simulink model "sm_metronome_sync_lots"  (R2026a)
settings: Solver=ode23t  StopTime=5.52*20  MaxStep=1e-2  AbsTol=1e-3  EnableMultiTasking=on
PreLoadFcn:
  | sm_metronome_sync_param
undefined symbols (not defined in the file): M1, M2, M3, M4, metronome, X, Y, Z
libraries: sm_lib x71, sm_metronome_lib x28, nesl_utility x3
(part 1 of 2)
CloseFcn:
  | try,close(h1_sm_metronome_sync),end
  | clear h1_sm_metronome_sync
  | try,close(h2_sm_metronome_sync),end
  | clear h2_sm_metronome_sync
  | try,close(h3_sm_metronome_sync),end
  | clear h3_sm_metronome_sync
  | try,close(h4_sm_metronome_sync),end
  | clear h4_sm_metronome_sync
  | 
  | 
  | clear simlog_sm_metronome_synch
  | clear logsout_sm_metronome_synch
Description:
  | Metronome Synchronization on Moving Platform, Multiple Rows
  | 
  | Copyright 2022-2026 The MathWorks, Inc.
settings Model: PacingRate=4  Creator=smiller  LastModifiedBy=smiller
settings DataIOCC: SaveFormat=StructureWithTime  SignalLoggingName=logsout_sm_metronome_sync
settings SimscapeCC: SimscapeNominalValues="[{\"value\":\"1\",\"unit\":\"A\"},{\"value\":\"1\",\"unit\":\"bar\"},{\"value\":\"1\",\"unit\":\"cm^2\"},{\"value\":\"1\",\"unit\":\"cm^3/s\"},{\"value\":\"1\",\"unit\":\"kJ/kg\"},{\"value\":\"1\",\"unit\":\"kW\"},{\"value\":\"1\",\"unit\":\"l\"},{\"value\":\"1\",\"unit\":\"N\"},{\"value\":\"1\",\"unit\":\"N*m\"},{\"value\":\"1\",\"unit\":\"V\"}]"  SimscapeLogSimulationStatistics=on  SimscapeLogName=simlog_sm_metronome_sync  SimscapeLogDataHistory=50000.0
settings ExplorerConfigSet: InternalSimMechanicsExplorerSettings="<ExplorerConfiguration><canonicalview>default</canonicalview><AnimationSetting><BasePlaybackSpeed>1.0</BasePlaybackSpeed><PlaybackSpeedFactor>4.0</PlaybackSpeedFactor></AnimationSetting><TilePanel><TileInfo><Tiles Columns=\"1\" Count=\"1\" Rows=\"1\"><Column Weight=\"1\"/><Row Weight=\"1\"/><Tile Height=\"1\" Width=\"1\" X=\"0\" Y=\"0\"/></Tiles></TileInfo><SceneInfo><SceneViewer><BGColor><R>1</R><G>1</G><B>1</B></BGColor><Camera><DoPerspective>off</DoPerspective><Position><X>0.415513055170568968</X><Y>-0.891822656871079644</Y><Z>0.234783488518173544</Z></Position><Center><X>-7.26516311720578896e-05</X><Y>0.00999648581965750446</Y><Z>0.116416456880806499</Z></Center><Up><X>-0.0260602284438559428</X><Y>0.118278053469418776</Y><Z>0.992638487346193754</Z></Up><ViewLimDist>1</ViewLimDist><YLim>0.195572453424284781</YLim><XLim>0.452734022015333248</XLim></Camera></SceneViewer></SceneInfo></TilePanel><MechEditorPanel><Cameras/><GfxPanelCameraMap/><VideoCreator><PlaybackSpeedRatio>1.0</PlaybackSpeedRatio><FrameRate>30</FrameRate><VideoFormat>Motion JPEG AVI</VideoFormat><FrameSize>auto</FrameSize></VideoCreator></MechEditorPanel></ExplorerConfiguration>"

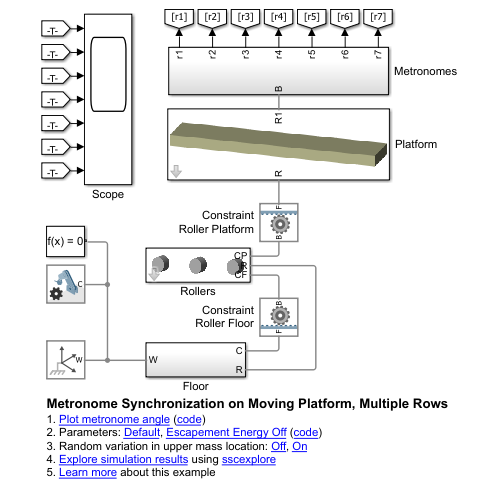
[thumbnail: Simulink's stored preview of the top-level diagram]
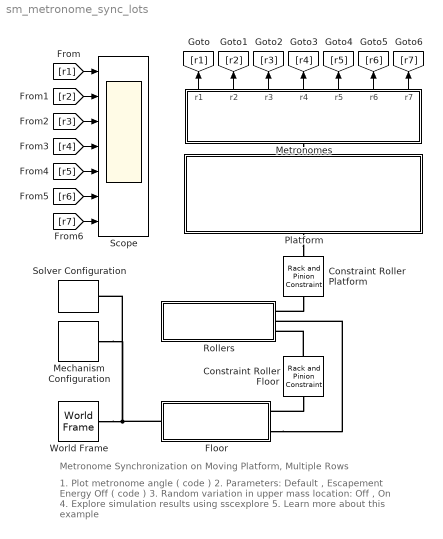
== system sm_metronome_sync_lots ==
  note: Metronome Synchronization on Moving Platform, Multiple Rows
  note: 1. Plot metronome angle ( code )
      | 2. Parameters: Default , Escapement Energy Off ( code )
      | 3. Random variation in upper mass location: Off , On
      | 4. Explore simulation results using sscexplore
      | 5. Learn more about this example
  Constraint Roller Floor : sm_lib/Gears and Couplings/Gears/Rack and Pinion Constraint  PinionRadius=metronome.roller_radius  PinionRadiusUnits=m  SensingForceTorqueDirection=FollowerOnBase  SensingForceTorqueResolutionFrame=BaseFrame  SenseForce=off  SenseTorque=off
  Constraint Roller Platform : sm_lib/Gears and Couplings/Gears/Rack and Pinion Constraint  PinionRadius=metronome.roller_radius  PinionRadiusUnits=m  SensingForceTorqueDirection=FollowerOnBase  SensingForceTorqueResolutionFrame=BaseFrame  SenseForce=off  SenseTorque=off
  Floor : Subsystem
  Mechanism Configuration : sm_lib/Utilities/Mechanism Configuration  UniformGravity=Constant  GravityVector=[0 0 -9.80665]  GravityVectorUnits=m/s^2  LinearizationDelta=0.001  JointModeTransitionNonlinearIterations=2
  Metronomes : Subsystem
  Platform : Subsystem  mask{t_unlock=10, platform_thk=metronome.platform_thickness, roller_rad=metronome.roller_radius}
      mask prompts: t_unlock "Time to Unlock Platform (sec)"; platform_thk "Platform Thickness"; roller_rad "Roller Radius (m)"
      mask Display: image('sm_metronome_sync_platform.png');
  Rollers : Subsystem  mask{roller_rad=metronome.roller_radius, roller_sep=metronome.roller_sep}
      mask prompts: roller_rad "Roller Radius (m)"; roller_sep "Roller Separation (m)"
      mask Display: image('sm_metronome_sync_rollers.png');
  Scope : Scope  NumInputPorts=7
      settings: TimeSpan=5.52/2  ActiveDisplayYMinimum=-1.09829  ActiveDisplayYMaximum=1.09791  DataLoggingVariableName=MetronomeAngles
  Solver Configuration : nesl_utility/Solver Configuration  PhysicalDomain=network_engine_domain  SubClassName=solver  LeftPortType=input  RightPortType=generic  Tones=[]  Harmonics=[]  SimulateNoise=off  Profile=off  UseLocalSampling=off  EnableSwitchedLinearOptims=on  FrequencyDomain=off  UseCCode=off  RelTol=0.001  AbsTol=1e-06  MinStep=1e-09  ToWorkspace=off  RevertToSquareIcSolve=off  NumHomotopyIterations=100  PhasorMode=off  PhasorModeNumHarmonics=1  ConsistencySolver=NEWTON_FTOL  CanonicalOrdering=UNORDERED  OptimizeIntermediates=UNOPTIMIZED  IndexReductionMethod=DerivativeReplacement  DoDC=off  ResidualTolerance=1e-09  ConsistencyTolSource=GLOBAL  ConsistencyAbsTol=0.001  ConsistencyRelTol=0.001  ConsistencyTolFactor=0.001  UseLocalSolver=off  LocalSolverChoice=NE_BACKWARD_EULER_ADVANCER  ResolveIndetEquations=on  FunctionEvalNumThread=1  LocalSolverSampleTime=0.001  DoFixedCost=off  MaxNonlinIter=3  MaxModeIter=2  ComputeImpulses=off  ImpulseIterations=2  LinearAlgebra=Sparse  LinearAlgebraNumThread=0  EquationFormulation=NE_TIME_EF  DelaysMemoryBudget=1024  AutomaticFiltering=on  FilteringTimeConstant=0.001  PartitionStorageMethod=AS_NEEDED  PartitionMemoryBudget=1024  PartitionMethod=FAST  MultibodyUseLocalSolver=off  MultibodyLocalSolverChoice=ODE1  MultibodyLocalSolverSampleTime=0.001
  World Frame : sm_lib/Frames and Transforms/World Frame
  wires:
  Metronomes/1(r1) -> [r1]
  Metronomes/2(r2) -> [r2]
  Metronomes/3(r3) -> [r3]
  Metronomes/4(r4) -> [r4]
  Metronomes/5(r5) -> [r5]
  Metronomes/6(r6) -> [r6]
  Metronomes/7(r7) -> [r7]
  [r1] -> Scope/1
  [r2] -> Scope/2
  [r3] -> Scope/3
  [r4] -> Scope/4
  [r5] -> Scope/5
  [r6] -> Scope/6
  [r7] -> Scope/7
  connections:
  World Frame/RConn1 -- Floor/LConn1 -- Solver Configuration/RConn1 -- Mechanism Configuration/RConn1
  Metronomes/LConn1 -- Platform/RConn1
  Constraint Roller Floor/LConn1 -- Rollers/RConn3
  Floor/RConn2 -- Rollers/RConn2
  Constraint Roller Platform/LConn1 -- Rollers/RConn1
  Constraint Roller Floor/RConn1 -- Floor/RConn1
  Platform/LConn1 -- Constraint Roller Platform/RConn1

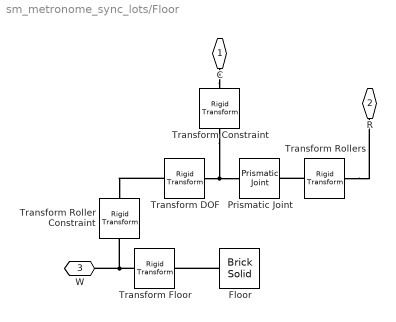
== system sm_metronome_sync_lots/Floor ==
  Floor : sm_lib/Body Elements/Brick Solid  BrickDimensions=[0.75 0.1 0.02]  BrickDimensionsUnits=m  ExportEntireGeometry=off  InertiaType=CalculateFromGeometry  BasedOnType=Density  Density=1000  DensityUnits=kg/m^3  Mass=1  MassUnits=kg  CenterOfMass=[0 0 0]  CenterOfMassUnits=m  MomentsOfInertia=[1 1 1]  MomentsOfInertiaUnits=kg*m^2  ProductsOfInertia=[0 0 0]  ProductsOfInertiaUnits=kg*m^2  GraphicType=FromGeometry  MarkerShape=Sphere  MarkerSize=10  GraphicVisPropType=SimpleVisualProperties  GraphicDiffuseColor=[0.5 0.5 0.5]  GraphicOpacity=1.0  GraphicSpecularColor=[0.5 0.5 0.5 1.0]  GraphicAmbientColor=[0.15 0.15 0.15 1.0]  GraphicEmissiveColor=[0.0 0.0 0.0 1.0]  GraphicShininess=75  DoExposeReferenceFrame=on  SerializedFrames=<Frames/>
  Prismatic Joint : sm_lib/Joints/Prismatic Joint  JointMode=Normal  CompositeWrenchDir=FollowerOnBase  CompositeWrenchFrame=BaseFrame  SenseConstraintForce=off  SenseConstraintTorque=off  SenseTotalForce=off  SenseTotalTorque=off  PositionTargetSpecify=off  PositionTargetPriority=High  PositionTargetValue=0  PositionTargetValueUnits=m  VelocityTargetSpecify=off  VelocityTargetPriority=High  VelocityTargetValue=0  VelocityTargetValueUnits=m/s  EquilibriumPosition=0  EquilibriumPositionUnits=m  SpringStiffness=0  SpringStiffnessUnits=N/m  DampingCoefficient=metronome.platform_damping  DampingCoefficientUnits=N/(m/s)  LowerLimitSpecify=off  LowerLimitBound=-1  LowerLimitBoundUnits=m  LowerLimitStiffness=1e6  LowerLimitStiffnessUnits=N/m  LowerLimitDamping=1e3  LowerLimitDampingUnits=N/(m/s)  LowerLimitTransitionRegionWidth=1e-4  LowerLimitTransitionRegionWidthUnits=m  UpperLimitSpecify=off  UpperLimitBound=1  UpperLimitBoundUnits=m  UpperLimitStiffness=1e6  UpperLimitStiffnessUnits=N/m  UpperLimitDamping=1e3  UpperLimitDampingUnits=N/(m/s)  UpperLimitTransitionRegionWidth=1e-4  UpperLimitTransitionRegionWidthUnits=m  TorqueActuationMode=NoTorque  MotionActuationMode=ComputedMotion  SensePosition=off  SenseVelocity=off  SenseAcceleration=off  SenseTorqueForce=off  SenseLowerLimitTorqueForce=off  SenseUpperLimitTorqueForce=off
  Transform Constraint : sm_lib/Frames and Transforms/Rigid Transform  RotationMethod=StandardAxis  FollAlignAxisA=+X  BaseAlignAxisA=+Y  FollAlignAxisB=+Y  BaseAlignAxisB=+Z  RotationStandardAxis=+Z  RotationAngle=0  RotationAngleUnits=deg  RotationArbitraryAxis=[0 0 1]  RotationSequenceAxes=FollowerAxes  RotationSequence=XYX  RotationSequenceAngles=[0 0 0]  RotationSequenceAnglesUnits=deg  RotationMatrix=[1 0 0; 0 1 0; 0 0 1]  Quaternion=[1 0 0 0]  TranslationMethod=StandardAxis  TranslationCartesianOffset=[0 0 0]  TranslationCartesianOffsetUnits=m  TranslationStandardAxis=+Y  TranslationStandardOffset=-metronome.roller_radius  TranslationStandardOffsetUnits=m  TranslationROffset=0  TranslationROffsetUnits=m  TranslationThetaOffset=0  TranslationThetaOffsetUnits=deg  TranslationZOffset=0  TranslationZOffsetUnits=m
  Transform DOF : sm_lib/Frames and Transforms/Rigid Transform  RotationMethod=StandardAxis  FollAlignAxisA=+X  BaseAlignAxisA=+Y  FollAlignAxisB=+Y  BaseAlignAxisB=+Z  RotationStandardAxis=+Y  RotationAngle=90  RotationAngleUnits=deg  RotationArbitraryAxis=[0 0 1]  RotationSequenceAxes=FollowerAxes  RotationSequence=XYX  RotationSequenceAngles=[0 0 0]  RotationSequenceAnglesUnits=deg  RotationMatrix=[1 0 0; 0 1 0; 0 0 1]  Quaternion=[1 0 0 0]  TranslationMethod=None  TranslationCartesianOffset=[0 0 0]  TranslationCartesianOffsetUnits=m  TranslationStandardAxis=+Z  TranslationStandardOffset=0  TranslationStandardOffsetUnits=m  TranslationROffset=0  TranslationROffsetUnits=m  TranslationThetaOffset=0  TranslationThetaOffsetUnits=deg  TranslationZOffset=0  TranslationZOffsetUnits=m
  Transform Floor : sm_lib/Frames and Transforms/Rigid Transform  RotationMethod=None  FollAlignAxisA=+X  BaseAlignAxisA=+Y  FollAlignAxisB=+Y  BaseAlignAxisB=+Z  RotationStandardAxis=+X  RotationAngle=90  RotationAngleUnits=deg  RotationArbitraryAxis=[0 0 1]  RotationSequenceAxes=FollowerAxes  RotationSequence=XYX  RotationSequenceAngles=[0 0 0]  RotationSequenceAnglesUnits=deg  RotationMatrix=[1 0 0; 0 1 0; 0 0 1]  Quaternion=[1 0 0 0]  TranslationMethod=StandardAxis  TranslationCartesianOffset=[0 0 0]  TranslationCartesianOffsetUnits=m  TranslationStandardAxis=+Z  TranslationStandardOffset=-0.01  TranslationStandardOffsetUnits=m  TranslationROffset=0  TranslationROffsetUnits=m  TranslationThetaOffset=0  TranslationThetaOffsetUnits=deg  TranslationZOffset=0  TranslationZOffsetUnits=m
  Transform Roller Constraint : sm_lib/Frames and Transforms/Rigid Transform  RotationMethod=StandardAxis  FollAlignAxisA=+X  BaseAlignAxisA=+Y  FollAlignAxisB=+Y  BaseAlignAxisB=+Z  RotationStandardAxis=+X  RotationAngle=90  RotationAngleUnits=deg  RotationArbitraryAxis=[0 0 1]  RotationSequenceAxes=FollowerAxes  RotationSequence=XYX  RotationSequenceAngles=[0 0 0]  RotationSequenceAnglesUnits=deg  RotationMatrix=[1 0 0; 0 1 0; 0 0 1]  Quaternion=[1 0 0 0]  TranslationMethod=StandardAxis  TranslationCartesianOffset=[0 0 0]  TranslationCartesianOffsetUnits=m  TranslationStandardAxis=+Z  TranslationStandardOffset=metronome.roller_radius  TranslationStandardOffsetUnits=m  TranslationROffset=0  TranslationROffsetUnits=m  TranslationThetaOffset=0  TranslationThetaOffsetUnits=deg  TranslationZOffset=0  TranslationZOffsetUnits=m
  Transform Rollers : sm_lib/Frames and Transforms/Rigid Transform  RotationMethod=RotationSequence  FollAlignAxisA=+X  BaseAlignAxisA=+Y  FollAlignAxisB=+Y  BaseAlignAxisB=+Z  RotationStandardAxis=+Y  RotationAngle=90  RotationAngleUnits=deg  RotationArbitraryAxis=[0 0 1]  RotationSequenceAxes=FollowerAxes  RotationSequence=YZY  RotationSequenceAngles=[-90 0 0]  RotationSequenceAnglesUnits=deg  RotationMatrix=[1 0 0; 0 1 0; 0 0 1]  Quaternion=[1 0 0 0]  TranslationMethod=None  TranslationCartesianOffset=[0 0 0]  TranslationCartesianOffsetUnits=m  TranslationStandardAxis=+Z  TranslationStandardOffset=0  TranslationStandardOffsetUnits=m  TranslationROffset=0  TranslationROffsetUnits=m  TranslationThetaOffset=0  TranslationThetaOffsetUnits=deg  TranslationZOffset=0  TranslationZOffsetUnits=m
  C : PMIOPort  Side=Right
  R : PMIOPort  Port=2  Side=Right
  W : PMIOPort  Port=3  Side=Left
  connections:
  Floor/RConn1 -- Transform Floor/RConn1
  Transform Rollers/LConn1 -- Prismatic Joint/RConn1
  Transform Floor/LConn1 -- Transform Roller Constraint/LConn1 -- W/RConn1
  Transform DOF/RConn1 -- Transform Constraint/LConn1 -- Prismatic Joint/LConn1
  Transform Rollers/RConn1 -- R/RConn1
  Transform DOF/LConn1 -- Transform Roller Constraint/RConn1
  C/RConn1 -- Transform Constraint/RConn1

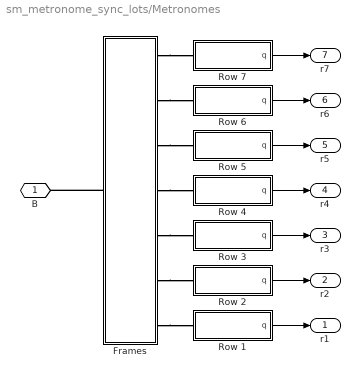
== system sm_metronome_sync_lots/Metronomes ==
  Frames : Subsystem
  Row 1 : Subsystem
  Row 2 : Subsystem
  Row 3 : Subsystem
  Row 4 : Subsystem
  Row 5 : Subsystem
  Row 6 : Subsystem
  Row 7 : Subsystem
  B : PMIOPort  Side=Left
  r1 : Outport
  r2 : Outport  Port=2
  r3 : Outport  Port=3
  r4 : Outport  Port=4
  r5 : Outport  Port=5
  r6 : Outport  Port=6
  r7 : Outport  Port=7
  wires:
  Row 1/1(q) -> r1/1
  Row 2/1(q) -> r2/1
  Row 4/1(q) -> r4/1
  Row 5/1(q) -> r5/1
  Row 3/1(q) -> r3/1
  Row 7/1(q) -> r7/1
  Row 6/1(q) -> r6/1
  connections:
  Frames/RConn3 -- Row 5/LConn1
  Frames/RConn7 -- Row 1/LConn1
  Frames/RConn6 -- Row 2/LConn1
  Frames/RConn5 -- Row 3/LConn1
  Frames/RConn2 -- Row 6/LConn1
  Frames/RConn4 -- Row 4/LConn1
  Frames/RConn1 -- Row 7/LConn1
  Frames/LConn1 -- B/RConn1

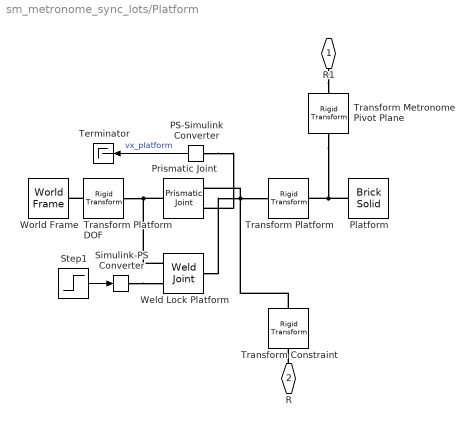
== system sm_metronome_sync_lots/Platform ==
  PS-Simulink Converter : nesl_utility/PS-Simulink Converter  PhysicalDomain=network_engine_domain  SubClassName=ps_output  LeftPortType=input  RightPortType=output  PseudoPeriodic=off  Frequencies=[]  VectorFormat=1-D array  Unit=inherit  AffineConversion=off
  Platform : sm_lib/Body Elements/Brick Solid  BrickDimensions=[0.75 0.75 platform_thk]  BrickDimensionsUnits=m  ExportEntireGeometry=on  InertiaType=CalculateFromGeometry  BasedOnType=Density  Density=10  DensityUnits=kg/m^3  Mass=1  MassUnits=kg  CenterOfMass=[0 0 0]  CenterOfMassUnits=m  MomentsOfInertia=[1 1 1]  MomentsOfInertiaUnits=kg*m^2  ProductsOfInertia=[0 0 0]  ProductsOfInertiaUnits=kg*m^2  GraphicType=FromGeometry  MarkerShape=Sphere  MarkerSize=10  GraphicVisPropType=SimpleVisualProperties  GraphicDiffuseColor=[0.84313726 0.84313726 0.6509804]  GraphicOpacity=1.0  GraphicSpecularColor=[0.5 0.5 0.5 1.0]  GraphicAmbientColor=[0.15 0.15 0.15 1.0]  GraphicEmissiveColor=[0.0 0.0 0.0 1.0]  GraphicShininess=75  DoExposeReferenceFrame=on  SerializedFrames=<Frames/>
  Prismatic Joint : sm_lib/Joints/Prismatic Joint  JointMode=Normal  CompositeWrenchDir=FollowerOnBase  CompositeWrenchFrame=BaseFrame  SenseConstraintForce=off  SenseConstraintTorque=off  SenseTotalForce=off  SenseTotalTorque=off  PositionTargetSpecify=off  PositionTargetPriority=High  PositionTargetValue=0  PositionTargetValueUnits=m  VelocityTargetSpecify=off  VelocityTargetPriority=High  VelocityTargetValue=0  VelocityTargetValueUnits=m/s  EquilibriumPosition=0  EquilibriumPositionUnits=m  SpringStiffness=100*0  SpringStiffnessUnits=N/m  DampingCoefficient=0  DampingCoefficientUnits=N/(m/s)  LowerLimitSpecify=off  LowerLimitBound=-1  LowerLimitBoundUnits=m  LowerLimitStiffness=1e6  LowerLimitStiffnessUnits=N/m  LowerLimitDamping=1e3  LowerLimitDampingUnits=N/(m/s)  LowerLimitTransitionRegionWidth=1e-4  LowerLimitTransitionRegionWidthUnits=m  UpperLimitSpecify=off  UpperLimitBound=1  UpperLimitBoundUnits=m  UpperLimitStiffness=1e6  UpperLimitStiffnessUnits=N/m  UpperLimitDamping=1e3  UpperLimitDampingUnits=N/(m/s)  UpperLimitTransitionRegionWidth=1e-4  UpperLimitTransitionRegionWidthUnits=m  TorqueActuationMode=NoTorque  MotionActuationMode=ComputedMotion  SensePosition=off  SenseVelocity=on  SenseAcceleration=off  SenseTorqueForce=off  SenseLowerLimitTorqueForce=off  SenseUpperLimitTorqueForce=off
  Simulink-PS Converter : nesl_utility/Simulink-PS Converter  PhysicalDomain=network_engine_domain  SubClassName=ps_input  LeftPortType=input  RightPortType=output  PseudoPeriodic=off  Frequencies=[]  NoiseDistribution=none  NoiseParameters=[]  Unit=1  AffineConversion=off  FilteringAndDerivatives=provide  SimscapeFilterOrder=1  InputFilterTimeConstant=0.001  UdotUserProvided=0
  Step1 : Step  Time=t_unlock  FinalValue=-1  SampleTime=0
  Terminator : Terminator
  Transform Constraint : sm_lib/Frames and Transforms/Rigid Transform  RotationMethod=StandardAxis  FollAlignAxisA=+X  BaseAlignAxisA=+Y  FollAlignAxisB=+Y  BaseAlignAxisB=+Z  RotationStandardAxis=+Z  RotationAngle=180  RotationAngleUnits=deg  RotationArbitraryAxis=[0 0 1]  RotationSequenceAxes=FollowerAxes  RotationSequence=XYX  RotationSequenceAngles=[0 0 0]  RotationSequenceAnglesUnits=deg  RotationMatrix=[1 0 0; 0 1 0; 0 0 1]  Quaternion=[1 0 0 0]  TranslationMethod=StandardAxis  TranslationCartesianOffset=[0 0 0]  TranslationCartesianOffsetUnits=m  TranslationStandardAxis=+Y  TranslationStandardOffset=-platform_thk/2  TranslationStandardOffsetUnits=m  TranslationROffset=0  TranslationROffsetUnits=m  TranslationThetaOffset=0  TranslationThetaOffsetUnits=deg  TranslationZOffset=0  TranslationZOffsetUnits=m
  Transform Metronome Pivot Plane : sm_lib/Frames and Transforms/Rigid Transform  RotationMethod=None  FollAlignAxisA=+X  BaseAlignAxisA=+Y  FollAlignAxisB=+Y  BaseAlignAxisB=+Z  RotationStandardAxis=+Z  RotationAngle=0.0  RotationAngleUnits=deg  RotationArbitraryAxis=[0 0 1]  RotationSequenceAxes=FollowerAxes  RotationSequence=XYX  RotationSequenceAngles=[0 0 0]  RotationSequenceAnglesUnits=deg  RotationMatrix=[1 0 0; 0 1 0; 0 0 1]  Quaternion=[1 0 0 0]  TranslationMethod=StandardAxis  TranslationCartesianOffset=[0 0 0]  TranslationCartesianOffsetUnits=m  TranslationStandardAxis=+Z  TranslationStandardOffset=platform_thk/2  TranslationStandardOffsetUnits=m  TranslationROffset=0  TranslationROffsetUnits=m  TranslationThetaOffset=0  TranslationThetaOffsetUnits=deg  TranslationZOffset=0  TranslationZOffsetUnits=m
  Transform Platform : sm_lib/Frames and Transforms/Rigid Transform  RotationMethod=RotationSequence  FollAlignAxisA=+X  BaseAlignAxisA=+Y  FollAlignAxisB=+Y  BaseAlignAxisB=+Z  RotationStandardAxis=+Z  RotationAngle=0.0  RotationAngleUnits=deg  RotationArbitraryAxis=[0 0 1]  RotationSequenceAxes=FollowerAxes  RotationSequence=YZX  RotationSequenceAngles=[90 90 0]  RotationSequenceAnglesUnits=deg  RotationMatrix=[1 0 0; 0 1 0; 0 0 1]  Quaternion=[1 0 0 0]  TranslationMethod=None  TranslationCartesianOffset=[0 0 0]  TranslationCartesianOffsetUnits=m  TranslationStandardAxis=+Z  TranslationStandardOffset=0  TranslationStandardOffsetUnits=m  TranslationROffset=0  TranslationROffsetUnits=m  TranslationThetaOffset=0  TranslationThetaOffsetUnits=deg  TranslationZOffset=0  TranslationZOffsetUnits=m
  Transform Platform DOF : sm_lib/Frames and Transforms/Rigid Transform  RotationMethod=RotationSequence  FollAlignAxisA=+X  BaseAlignAxisA=+Y  FollAlignAxisB=+Y  BaseAlignAxisB=+Z  RotationStandardAxis=+Z  RotationAngle=0.0  RotationAngleUnits=deg  RotationArbitraryAxis=[0 0 1]  RotationSequenceAxes=FollowerAxes  RotationSequence=YZX  RotationSequenceAngles=[90 90 0]  RotationSequenceAnglesUnits=deg  RotationMatrix=[1 0 0; 0 1 0; 0 0 1]  Quaternion=[1 0 0 0]  TranslationMethod=StandardAxis  TranslationCartesianOffset=[0 0 0]  TranslationCartesianOffsetUnits=m  TranslationStandardAxis=+Z  TranslationStandardOffset=roller_rad*2+platform_thk/2  TranslationStandardOffsetUnits=m  TranslationROffset=0  TranslationROffsetUnits=m  TranslationThetaOffset=0  TranslationThetaOffsetUnits=deg  TranslationZOffset=0  TranslationZOffsetUnits=m
  Weld Lock Platform : sm_lib/Joints/Weld Joint  JointMode=ProvidedByInput  CompositeWrenchDir=FollowerOnBase  CompositeWrenchFrame=BaseFrame  SenseConstraintForce=off  SenseConstraintTorque=off  SenseTotalForce=off  SenseTotalTorque=off
  World Frame : sm_lib/Frames and Transforms/World Frame
  R1 : PMIOPort  Side=Right
  R : PMIOPort  Port=2  Side=Left
  wires:
  Step1/1 -> Simulink-PS Converter/1
  PS-Simulink Converter/1 -> Terminator/1  "vx_platform"
  connections:
  Prismatic Joint/RConn1 -- Weld Lock Platform/RConn1 -- Transform Constraint/LConn1 -- Transform Platform/RConn1
  Platform/RConn1 -- Transform Metronome Pivot Plane/LConn1 -- Transform Platform/LConn1
  Transform Platform DOF/RConn1 -- Prismatic Joint/LConn1 -- Weld Lock Platform/LConn1
  Transform Platform DOF/LConn1 -- World Frame/RConn1
  Simulink-PS Converter/RConn1 -- Weld Lock Platform/LConn2
  R1/RConn1 -- Transform Metronome Pivot Plane/RConn1
  PS-Simulink Converter/LConn1 -- Prismatic Joint/RConn2
  R/RConn1 -- Transform Constraint/RConn1

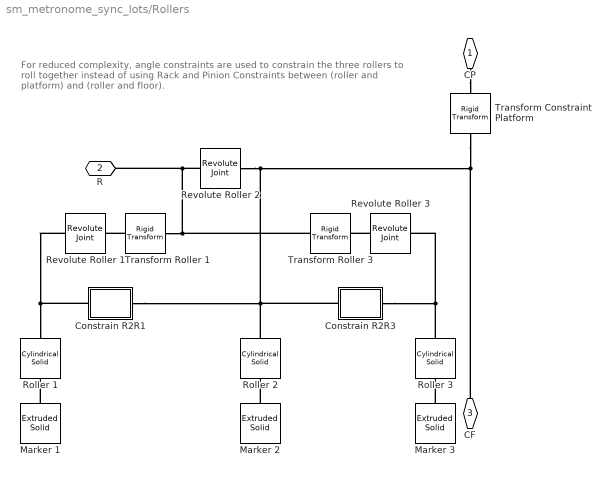
== system sm_metronome_sync_lots/Rollers ==
  note: For reduced complexity, angle constraints are used to constrain the three rollers to roll together instead of using Rack and Pinion Constraints between (roller and platform) and (roller and floor).
  Constrain R2R1 : Subsystem
  Constrain R2R3 : Subsystem
  Marker 1 : sm_lib/Body Elements/Extruded Solid  ExtrusionType=Regular  PolygonNumSides=6  PolygonOuterRadius=roller_rad*0.9  PolygonOuterRadiusUnits=m  ExportEntireGeometry=off  ExtrusionCrossSection=[1 1; -1 1; -1 -1; 1 -1]  ExtrusionCrossSectionUnits=m  ExportConvexHullGeometry=off  ExtrusionLength=1e-3  ExtrusionLengthUnits=m  InertiaType=CalculateFromGeometry  BasedOnType=Mass  Density=1000  DensityUnits=kg/m^3  Mass=0  MassUnits=kg  CenterOfMass=[0 0 0]  CenterOfMassUnits=m  MomentsOfInertia=[1 1 1]  MomentsOfInertiaUnits=kg*m^2  ProductsOfInertia=[0 0 0]  ProductsOfInertiaUnits=kg*m^2  GraphicType=FromGeometry  MarkerShape=Sphere  MarkerSize=10  GraphicVisPropType=SimpleVisualProperties  GraphicDiffuseColor=[0.0 0.2 0.4]  GraphicOpacity=1.0  GraphicSpecularColor=[0.5 0.5 0.5 1.0]  GraphicAmbientColor=[0.15 0.15 0.15 1.0]  GraphicEmissiveColor=[0.0 0.0 0.0 1.0]  GraphicShininess=75  DoExposeReferenceFrame=on  SerializedFrames=<Frames/>
  Marker 2 : sm_lib/Body Elements/Extruded Solid  ExtrusionType=Regular  PolygonNumSides=6  PolygonOuterRadius=roller_rad*0.9  PolygonOuterRadiusUnits=m  ExportEntireGeometry=off  ExtrusionCrossSection=[1 1; -1 1; -1 -1; 1 -1]  ExtrusionCrossSectionUnits=m  ExportConvexHullGeometry=off  ExtrusionLength=1e-3  ExtrusionLengthUnits=m  InertiaType=CalculateFromGeometry  BasedOnType=Mass  Density=1000  DensityUnits=kg/m^3  Mass=0  MassUnits=kg  CenterOfMass=[0 0 0]  CenterOfMassUnits=m  MomentsOfInertia=[1 1 1]  MomentsOfInertiaUnits=kg*m^2  ProductsOfInertia=[0 0 0]  ProductsOfInertiaUnits=kg*m^2  GraphicType=FromGeometry  MarkerShape=Sphere  MarkerSize=10  GraphicVisPropType=SimpleVisualProperties  GraphicDiffuseColor=[0.0 0.2 0.4]  GraphicOpacity=1.0  GraphicSpecularColor=[0.5 0.5 0.5 1.0]  GraphicAmbientColor=[0.15 0.15 0.15 1.0]  GraphicEmissiveColor=[0.0 0.0 0.0 1.0]  GraphicShininess=75  DoExposeReferenceFrame=on  SerializedFrames=<Frames/>
  Marker 3 : sm_lib/Body Elements/Extruded Solid  ExtrusionType=Regular  PolygonNumSides=6  PolygonOuterRadius=roller_rad*0.9  PolygonOuterRadiusUnits=m  ExportEntireGeometry=off  ExtrusionCrossSection=[1 1; -1 1; -1 -1; 1 -1]  ExtrusionCrossSectionUnits=m  ExportConvexHullGeometry=off  ExtrusionLength=1e-3  ExtrusionLengthUnits=m  InertiaType=CalculateFromGeometry  BasedOnType=Mass  Density=1000  DensityUnits=kg/m^3  Mass=0  MassUnits=kg  CenterOfMass=[0 0 0]  CenterOfMassUnits=m  MomentsOfInertia=[1 1 1]  MomentsOfInertiaUnits=kg*m^2  ProductsOfInertia=[0 0 0]  ProductsOfInertiaUnits=kg*m^2  GraphicType=FromGeometry  MarkerShape=Sphere  MarkerSize=10  GraphicVisPropType=SimpleVisualProperties  GraphicDiffuseColor=[0.0 0.2 0.4]  GraphicOpacity=1.0  GraphicSpecularColor=[0.5 0.5 0.5 1.0]  GraphicAmbientColor=[0.15 0.15 0.15 1.0]  GraphicEmissiveColor=[0.0 0.0 0.0 1.0]  GraphicShininess=75  DoExposeReferenceFrame=on  SerializedFrames=<Frames/>
  Revolute Roller 1 : sm_lib/Joints/Revolute Joint  JointMode=Normal  CompositeWrenchDir=FollowerOnBase  CompositeWrenchFrame=BaseFrame  SenseConstraintForce=off  SenseConstraintTorque=off  SenseTotalForce=off  SenseTotalTorque=off  PositionTargetSpecify=off  PositionTargetPriority=High  PositionTargetValue=0  PositionTargetValueUnits=deg  VelocityTargetSpecify=off  VelocityTargetPriority=High  VelocityTargetValue=0  VelocityTargetValueUnits=deg/s  EquilibriumPosition=0  EquilibriumPositionUnits=deg  SpringStiffness=0  SpringStiffnessUnits=N*m/deg  DampingCoefficient=0  DampingCoefficientUnits=N*m/(deg/s)  LowerLimitSpecify=off  LowerLimitBound=-90  LowerLimitBoundUnits=deg  LowerLimitStiffness=1e4  LowerLimitStiffnessUnits=N*m/deg  LowerLimitDamping=10  LowerLimitDampingUnits=N*m/(deg/s)  LowerLimitTransitionRegionWidth=0.1  LowerLimitTransitionRegionWidthUnits=deg  UpperLimitSpecify=off  UpperLimitBound=90  UpperLimitBoundUnits=deg  UpperLimitStiffness=1e4  UpperLimitStiffnessUnits=N*m/deg  UpperLimitDamping=10  UpperLimitDampingUnits=N*m/(deg/s)  UpperLimitTransitionRegionWidth=0.1  UpperLimitTransitionRegionWidthUnits=deg  TorqueActuationMode=NoTorque  MotionActuationMode=ComputedMotion  SensePosition=off  SenseVelocity=off  SenseAcceleration=off  SenseTorqueForce=off  SenseLowerLimitTorqueForce=off  SenseUpperLimitTorqueForce=off
  Revolute Roller 2 : sm_lib/Joints/Revolute Joint  JointMode=Normal  CompositeWrenchDir=FollowerOnBase  CompositeWrenchFrame=BaseFrame  SenseConstraintForce=off  SenseConstraintTorque=off  SenseTotalForce=off  SenseTotalTorque=off  PositionTargetSpecify=off  PositionTargetPriority=High  PositionTargetValue=0  PositionTargetValueUnits=deg  VelocityTargetSpecify=off  VelocityTargetPriority=High  VelocityTargetValue=0  VelocityTargetValueUnits=deg/s  EquilibriumPosition=0  EquilibriumPositionUnits=deg  SpringStiffness=0  SpringStiffnessUnits=N*m/deg  DampingCoefficient=0  DampingCoefficientUnits=N*m/(deg/s)  LowerLimitSpecify=off  LowerLimitBound=-90  LowerLimitBoundUnits=deg  LowerLimitStiffness=1e4  LowerLimitStiffnessUnits=N*m/deg  LowerLimitDamping=10  LowerLimitDampingUnits=N*m/(deg/s)  LowerLimitTransitionRegionWidth=0.1  LowerLimitTransitionRegionWidthUnits=deg  UpperLimitSpecify=off  UpperLimitBound=90  UpperLimitBoundUnits=deg  UpperLimitStiffness=1e4  UpperLimitStiffnessUnits=N*m/deg  UpperLimitDamping=10  UpperLimitDampingUnits=N*m/(deg/s)  UpperLimitTransitionRegionWidth=0.1  UpperLimitTransitionRegionWidthUnits=deg  TorqueActuationMode=NoTorque  MotionActuationMode=ComputedMotion  SensePosition=off  SenseVelocity=off  SenseAcceleration=off  SenseTorqueForce=off  SenseLowerLimitTorqueForce=off  SenseUpperLimitTorqueForce=off
  Revolute Roller 3 : sm_lib/Joints/Revolute Joint  JointMode=Normal  CompositeWrenchDir=FollowerOnBase  CompositeWrenchFrame=BaseFrame  SenseConstraintForce=off  SenseConstraintTorque=off  SenseTotalForce=off  SenseTotalTorque=off  PositionTargetSpecify=off  PositionTargetPriority=High  PositionTargetValue=0  PositionTargetValueUnits=deg  VelocityTargetSpecify=off  VelocityTargetPriority=High  VelocityTargetValue=0  VelocityTargetValueUnits=deg/s  EquilibriumPosition=0  EquilibriumPositionUnits=deg  SpringStiffness=0  SpringStiffnessUnits=N*m/deg  DampingCoefficient=0  DampingCoefficientUnits=N*m/(deg/s)  LowerLimitSpecify=off  LowerLimitBound=-90  LowerLimitBoundUnits=deg  LowerLimitStiffness=1e4  LowerLimitStiffnessUnits=N*m/deg  LowerLimitDamping=10  LowerLimitDampingUnits=N*m/(deg/s)  LowerLimitTransitionRegionWidth=0.1  LowerLimitTransitionRegionWidthUnits=deg  UpperLimitSpecify=off  UpperLimitBound=90  UpperLimitBoundUnits=deg  UpperLimitStiffness=1e4  UpperLimitStiffnessUnits=N*m/deg  UpperLimitDamping=10  UpperLimitDampingUnits=N*m/(deg/s)  UpperLimitTransitionRegionWidth=0.1  UpperLimitTransitionRegionWidthUnits=deg  TorqueActuationMode=NoTorque  MotionActuationMode=ComputedMotion  SensePosition=off  SenseVelocity=off  SenseAcceleration=off  SenseTorqueForce=off  SenseLowerLimitTorqueForce=off  SenseUpperLimitTorqueForce=off
  Roller 1 : sm_lib/Body Elements/Cylindrical Solid  CylinderRadius=roller_rad  CylinderRadiusUnits=m  CylinderLength=0.08  CylinderLengthUnits=m  ExportEntireGeometry=off  InertiaType=CalculateFromGeometry  BasedOnType=Density  Density=1  DensityUnits=kg/m^3  Mass=1  MassUnits=kg  CenterOfMass=[0 0 0]  CenterOfMassUnits=m  MomentsOfInertia=[1 1 1]  MomentsOfInertiaUnits=kg*m^2  ProductsOfInertia=[0 0 0]  ProductsOfInertiaUnits=kg*m^2  GraphicType=FromGeometry  MarkerShape=Sphere  MarkerSize=10  GraphicVisPropType=SimpleVisualProperties  GraphicDiffuseColor=[0.8 0.8 0.8]  GraphicOpacity=1.0  GraphicSpecularColor=[0.5 0.5 0.5 1.0]  GraphicAmbientColor=[0.15 0.15 0.15 1.0]  GraphicEmissiveColor=[0.0 0.0 0.0 1.0]  GraphicShininess=75  DoExposeReferenceFrame=on  SerializedFrames=<Frames><Frame><Id>Frame1</Id><Value><Name>F</Name><Origin><Source>GeometricFeature</Source><FeatureName>top surface</FeatureName></Origin><PrimaryAxis><DefinedDirection>+Z</DefinedDirection><Source>ReferenceFrame</Source><SourceDirection>+Z</SourceDirection><FeatureName></FeatureName></PrimaryAxis><SecondaryAxis><DefinedDirection>+X</DefinedDirection><Source>ReferenceFrame</Source><SourceDirection>+X</SourceDirection><FeatureName></FeatureName></SecondaryAxis></Value></Frame></Frames>
  Roller 2 : sm_lib/Body Elements/Cylindrical Solid  CylinderRadius=roller_rad  CylinderRadiusUnits=m  CylinderLength=0.08  CylinderLengthUnits=m  ExportEntireGeometry=off  InertiaType=CalculateFromGeometry  BasedOnType=Density  Density=1  DensityUnits=kg/m^3  Mass=1  MassUnits=kg  CenterOfMass=[0 0 0]  CenterOfMassUnits=m  MomentsOfInertia=[1 1 1]  MomentsOfInertiaUnits=kg*m^2  ProductsOfInertia=[0 0 0]  ProductsOfInertiaUnits=kg*m^2  GraphicType=FromGeometry  MarkerShape=Sphere  MarkerSize=10  GraphicVisPropType=SimpleVisualProperties  GraphicDiffuseColor=[0.8 0.8 0.8]  GraphicOpacity=1.0  GraphicSpecularColor=[0.5 0.5 0.5 1.0]  GraphicAmbientColor=[0.15 0.15 0.15 1.0]  GraphicEmissiveColor=[0.0 0.0 0.0 1.0]  GraphicShininess=75  DoExposeReferenceFrame=on  SerializedFrames=<Frames><Frame><Id>Frame1</Id><Value><Name>F</Name><Origin><Source>GeometricFeature</Source><FeatureName>top surface</FeatureName></Origin><PrimaryAxis><DefinedDirection>+Z</DefinedDirection><Source>ReferenceFrame</Source><SourceDirection>+Z</SourceDirection><FeatureName></FeatureName></PrimaryAxis><SecondaryAxis><DefinedDirection>+X</DefinedDirection><Source>ReferenceFrame</Source><SourceDirection>+X</SourceDirection><FeatureName></FeatureName></SecondaryAxis></Value></Frame></Frames>
  Roller 3 : sm_lib/Body Elements/Cylindrical Solid  CylinderRadius=roller_rad  CylinderRadiusUnits=m  CylinderLength=0.08  CylinderLengthUnits=m  ExportEntireGeometry=off  InertiaType=CalculateFromGeometry  BasedOnType=Density  Density=1  DensityUnits=kg/m^3  Mass=1  MassUnits=kg  CenterOfMass=[0 0 0]  CenterOfMassUnits=m  MomentsOfInertia=[1 1 1]  MomentsOfInertiaUnits=kg*m^2  ProductsOfInertia=[0 0 0]  ProductsOfInertiaUnits=kg*m^2  GraphicType=FromGeometry  MarkerShape=Sphere  MarkerSize=10  GraphicVisPropType=SimpleVisualProperties  GraphicDiffuseColor=[0.8 0.8 0.8]  GraphicOpacity=1.0  GraphicSpecularColor=[0.5 0.5 0.5 1.0]  GraphicAmbientColor=[0.15 0.15 0.15 1.0]  GraphicEmissiveColor=[0.0 0.0 0.0 1.0]  GraphicShininess=75  DoExposeReferenceFrame=on  SerializedFrames=<Frames><Frame><Id>Frame1</Id><Value><Name>F</Name><Origin><Source>GeometricFeature</Source><FeatureName>top surface</FeatureName></Origin><PrimaryAxis><DefinedDirection>+Z</DefinedDirection><Source>ReferenceFrame</Source><SourceDirection>+Z</SourceDirection><FeatureName></FeatureName></PrimaryAxis><SecondaryAxis><DefinedDirection>+X</DefinedDirection><Source>ReferenceFrame</Source><SourceDirection>+X</SourceDirection><FeatureName></FeatureName></SecondaryAxis></Value></Frame></Frames>
  Transform Constraint Platform : sm_lib/Frames and Transforms/Rigid Transform  RotationMethod=StandardAxis  FollAlignAxisA=+X  BaseAlignAxisA=+Y  FollAlignAxisB=+Y  BaseAlignAxisB=+Z  RotationStandardAxis=+X  RotationAngle=180  RotationAngleUnits=deg  RotationArbitraryAxis=[0 0 1]  RotationSequenceAxes=FollowerAxes  RotationSequence=XYX  RotationSequenceAngles=[0 0 0]  RotationSequenceAnglesUnits=deg  RotationMatrix=[1 0 0; 0 1 0; 0 0 1]  Quaternion=[1 0 0 0]  TranslationMethod=None  TranslationCartesianOffset=[0 0 0]  TranslationCartesianOffsetUnits=m  TranslationStandardAxis=+Z  TranslationStandardOffset=0  TranslationStandardOffsetUnits=m  TranslationROffset=0  TranslationROffsetUnits=m  TranslationThetaOffset=0  TranslationThetaOffsetUnits=deg  TranslationZOffset=0  TranslationZOffsetUnits=m
  Transform Roller 1 : sm_lib/Frames and Transforms/Rigid Transform  RotationMethod=None  FollAlignAxisA=+X  BaseAlignAxisA=+Y  FollAlignAxisB=+Y  BaseAlignAxisB=+Z  RotationStandardAxis=+Z  RotationAngle=0.0  RotationAngleUnits=deg  RotationArbitraryAxis=[0 0 1]  RotationSequenceAxes=FollowerAxes  RotationSequence=XYX  RotationSequenceAngles=[0 0 0]  RotationSequenceAnglesUnits=deg  RotationMatrix=[1 0 0; 0 1 0; 0 0 1]  Quaternion=[1 0 0 0]  TranslationMethod=StandardAxis  TranslationCartesianOffset=[0 0 0]  TranslationCartesianOffsetUnits=m  TranslationStandardAxis=+X  TranslationStandardOffset=roller_sep  TranslationStandardOffsetUnits=m  TranslationROffset=0  TranslationROffsetUnits=m  TranslationThetaOffset=0  TranslationThetaOffsetUnits=deg  TranslationZOffset=0  TranslationZOffsetUnits=m
  Transform Roller 3 : sm_lib/Frames and Transforms/Rigid Transform  RotationMethod=None  FollAlignAxisA=+X  BaseAlignAxisA=+Y  FollAlignAxisB=+Y  BaseAlignAxisB=+Z  RotationStandardAxis=+Z  RotationAngle=0.0  RotationAngleUnits=deg  RotationArbitraryAxis=[0 0 1]  RotationSequenceAxes=FollowerAxes  RotationSequence=XYX  RotationSequenceAngles=[0 0 0]  RotationSequenceAnglesUnits=deg  RotationMatrix=[1 0 0; 0 1 0; 0 0 1]  Quaternion=[1 0 0 0]  TranslationMethod=StandardAxis  TranslationCartesianOffset=[0 0 0]  TranslationCartesianOffsetUnits=m  TranslationStandardAxis=+X  TranslationStandardOffset=roller_sep  TranslationStandardOffsetUnits=m  TranslationROffset=0  TranslationROffsetUnits=m  TranslationThetaOffset=0  TranslationThetaOffsetUnits=deg  TranslationZOffset=0  TranslationZOffsetUnits=m
  CP : PMIOPort  Side=Right
  R : PMIOPort  Port=2  Side=Right
  CF : PMIOPort  Port=3  Side=Right
  connections:
  CP/RConn1 -- Transform Constraint Platform/RConn1
  Revolute Roller 2/RConn1 -- Roller 2/RConn1 -- Constrain R2R1/RConn1 -- Constrain R2R3/RConn1 -- CF/RConn1 -- Transform Constraint Platform/LConn1
  Constrain R2R3/LConn1 -- Roller 3/RConn1 -- Revolute Roller 3/RConn1
  Transform Roller 1/LConn1 -- Revolute Roller 1/LConn1
  Revolute Roller 2/LConn1 -- Transform Roller 3/LConn1 -- Transform Roller 1/RConn1 -- R/RConn1
  Revolute Roller 1/RConn1 -- Constrain R2R1/LConn1 -- Roller 1/RConn1
  Revolute Roller 3/LConn1 -- Transform Roller 3/RConn1
  Marker 1/RConn1 -- Roller 1/LConn1
  Marker 2/RConn1 -- Roller 2/LConn1
  Marker 3/RConn1 -- Roller 3/LConn1

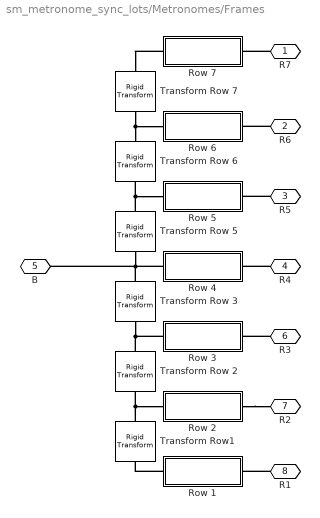
== system sm_metronome_sync_lots/Metronomes/Frames ==
  Row 1 : Subsystem
  Row 2 : Subsystem
  Row 3 : Subsystem
  Row 4 : Subsystem
  Row 5 : Subsystem
  Row 6 : Subsystem
  Row 7 : Subsystem
  Transform Row 2 : sm_lib/Frames and Transforms/Rigid Transform  RotationMethod=None  FollAlignAxisA=+X  BaseAlignAxisA=+Y  FollAlignAxisB=+Y  BaseAlignAxisB=+Z  RotationStandardAxis=+X  RotationAngle=90  RotationAngleUnits=deg  RotationArbitraryAxis=[0 0 1]  RotationSequenceAxes=FollowerAxes  RotationSequence=XYX  RotationSequenceAngles=[0 0 0]  RotationSequenceAnglesUnits=deg  RotationMatrix=[1 0 0; 0 1 0; 0 0 1]  Quaternion=[1 0 0 0]  TranslationMethod=StandardAxis  TranslationCartesianOffset=[-0.1 0 0]  TranslationCartesianOffsetUnits=m  TranslationStandardAxis=+Y  TranslationStandardOffset=-0.1  TranslationStandardOffsetUnits=m  TranslationROffset=0  TranslationROffsetUnits=m  TranslationThetaOffset=0  TranslationThetaOffsetUnits=deg  TranslationZOffset=0  TranslationZOffsetUnits=m
  Transform Row 3 : sm_lib/Frames and Transforms/Rigid Transform  RotationMethod=None  FollAlignAxisA=+X  BaseAlignAxisA=+Y  FollAlignAxisB=+Y  BaseAlignAxisB=+Z  RotationStandardAxis=+X  RotationAngle=90  RotationAngleUnits=deg  RotationArbitraryAxis=[0 0 1]  RotationSequenceAxes=FollowerAxes  RotationSequence=XYX  RotationSequenceAngles=[0 0 0]  RotationSequenceAnglesUnits=deg  RotationMatrix=[1 0 0; 0 1 0; 0 0 1]  Quaternion=[1 0 0 0]  TranslationMethod=StandardAxis  TranslationCartesianOffset=[-0.1 0 0]  TranslationCartesianOffsetUnits=m  TranslationStandardAxis=+Y  TranslationStandardOffset=-0.1  TranslationStandardOffsetUnits=m  TranslationROffset=0  TranslationROffsetUnits=m  TranslationThetaOffset=0  TranslationThetaOffsetUnits=deg  TranslationZOffset=0  TranslationZOffsetUnits=m
  Transform Row 5 : sm_lib/Frames and Transforms/Rigid Transform  RotationMethod=None  FollAlignAxisA=+X  BaseAlignAxisA=+Y  FollAlignAxisB=+Y  BaseAlignAxisB=+Z  RotationStandardAxis=+X  RotationAngle=90  RotationAngleUnits=deg  RotationArbitraryAxis=[0 0 1]  RotationSequenceAxes=FollowerAxes  RotationSequence=XYX  RotationSequenceAngles=[0 0 0]  RotationSequenceAnglesUnits=deg  RotationMatrix=[1 0 0; 0 1 0; 0 0 1]  Quaternion=[1 0 0 0]  TranslationMethod=StandardAxis  TranslationCartesianOffset=[-0.1 0 0]  TranslationCartesianOffsetUnits=m  TranslationStandardAxis=-Y  TranslationStandardOffset=-0.1  TranslationStandardOffsetUnits=m  TranslationROffset=0  TranslationROffsetUnits=m  TranslationThetaOffset=0  TranslationThetaOffsetUnits=deg  TranslationZOffset=0  TranslationZOffsetUnits=m
  Transform Row 6 : sm_lib/Frames and Transforms/Rigid Transform  RotationMethod=None  FollAlignAxisA=+X  BaseAlignAxisA=+Y  FollAlignAxisB=+Y  BaseAlignAxisB=+Z  RotationStandardAxis=+X  RotationAngle=90  RotationAngleUnits=deg  RotationArbitraryAxis=[0 0 1]  RotationSequenceAxes=FollowerAxes  RotationSequence=XYX  RotationSequenceAngles=[0 0 0]  RotationSequenceAnglesUnits=deg  RotationMatrix=[1 0 0; 0 1 0; 0 0 1]  Quaternion=[1 0 0 0]  TranslationMethod=StandardAxis  TranslationCartesianOffset=[-0.1 0 0]  TranslationCartesianOffsetUnits=m  TranslationStandardAxis=-Y  TranslationStandardOffset=-0.1  TranslationStandardOffsetUnits=m  TranslationROffset=0  TranslationROffsetUnits=m  TranslationThetaOffset=0  TranslationThetaOffsetUnits=deg  TranslationZOffset=0  TranslationZOffsetUnits=m
  Transform Row 7 : sm_lib/Frames and Transforms/Rigid Transform  RotationMethod=None  FollAlignAxisA=+X  BaseAlignAxisA=+Y  FollAlignAxisB=+Y  BaseAlignAxisB=+Z  RotationStandardAxis=+X  RotationAngle=90  RotationAngleUnits=deg  RotationArbitraryAxis=[0 0 1]  RotationSequenceAxes=FollowerAxes  RotationSequence=XYX  RotationSequenceAngles=[0 0 0]  RotationSequenceAnglesUnits=deg  RotationMatrix=[1 0 0; 0 1 0; 0 0 1]  Quaternion=[1 0 0 0]  TranslationMethod=StandardAxis  TranslationCartesianOffset=[-0.1 0 0]  TranslationCartesianOffsetUnits=m  TranslationStandardAxis=-Y  TranslationStandardOffset=-0.1  TranslationStandardOffsetUnits=m  TranslationROffset=0  TranslationROffsetUnits=m  TranslationThetaOffset=0  TranslationThetaOffsetUnits=deg  TranslationZOffset=0  TranslationZOffsetUnits=m
  Transform Row1 : sm_lib/Frames and Transforms/Rigid Transform  RotationMethod=None  FollAlignAxisA=+X  BaseAlignAxisA=+Y  FollAlignAxisB=+Y  BaseAlignAxisB=+Z  RotationStandardAxis=+X  RotationAngle=90  RotationAngleUnits=deg  RotationArbitraryAxis=[0 0 1]  RotationSequenceAxes=FollowerAxes  RotationSequence=XYX  RotationSequenceAngles=[0 0 0]  RotationSequenceAnglesUnits=deg  RotationMatrix=[1 0 0; 0 1 0; 0 0 1]  Quaternion=[1 0 0 0]  TranslationMethod=StandardAxis  TranslationCartesianOffset=[-0.1 0 0]  TranslationCartesianOffsetUnits=m  TranslationStandardAxis=+Y  TranslationStandardOffset=-0.1  TranslationStandardOffsetUnits=m  TranslationROffset=0  TranslationROffsetUnits=m  TranslationThetaOffset=0  TranslationThetaOffsetUnits=deg  TranslationZOffset=0  TranslationZOffsetUnits=m
  R7 : PMIOPort  Side=Right
  R6 : PMIOPort  Port=2  Side=Right
  R5 : PMIOPort  Port=3  Side=Right
  R4 : PMIOPort  Port=4  Side=Right
  B : PMIOPort  Port=5  Side=Left
  R3 : PMIOPort  Port=6  Side=Right
  R2 : PMIOPort  Port=7  Side=Right
  R1 : PMIOPort  Port=8  Side=Right
  connections:
  Transform Row 7/LConn1 -- Transform Row 6/RConn1 -- Row 6/LConn1
  R7/RConn1 -- Row 7/RConn1
  Transform Row 3/LConn1 -- Row 4/LConn1 -- Transform Row 5/LConn1 -- B/RConn1
  Transform Row 2/LConn1 -- Transform Row 3/RConn1 -- Row 3/LConn1
  Transform Row 5/RConn1 -- Row 5/LConn1 -- Transform Row 6/LConn1
  Row 1/LConn1 -- Transform Row1/RConn1
  Transform Row1/LConn1 -- Row 2/LConn1 -- Transform Row 2/RConn1
  R5/RConn1 -- Row 5/RConn1
  Row 7/LConn1 -- Transform Row 7/RConn1
  R3/RConn1 -- Row 3/RConn1
  Row 2/RConn1 -- R2/RConn1
  R1/RConn1 -- Row 1/RConn1
  R6/RConn1 -- Row 6/RConn1
  R4/RConn1 -- Row 4/RConn1

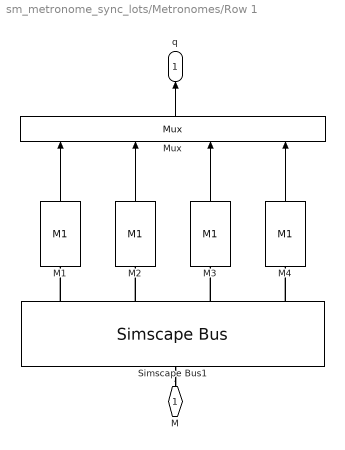
== system sm_metronome_sync_lots/Metronomes/Row 1 ==
  M1 : sm_metronome_lib/M1  pivot_h=metronome.pivot_h  len=metronome.stem_length  upper_len=metronome.stem_upper  upper_len_var=metronome.stem_upper_var  upper_m=metronome.upper_mass  lower_m=metronome.lower_mass  b_pivot=metronome.b_pivot  esc_torque=metronome.esc_torque  t0_ang=-15 + (30)*rand(1,1)  t0_vel=metronome.initial_speed(1)
  M2 : sm_metronome_lib/M1  pivot_h=metronome.pivot_h  len=metronome.stem_length  upper_len=metronome.stem_upper  upper_len_var=metronome.stem_upper_var  upper_m=metronome.upper_mass  lower_m=metronome.lower_mass  b_pivot=metronome.b_pivot  esc_torque=metronome.esc_torque  t0_ang=-15 + (30)*rand(1,1)  t0_vel=metronome.initial_speed(2)
  M3 : sm_metronome_lib/M1  pivot_h=metronome.pivot_h  len=metronome.stem_length  upper_len=metronome.stem_upper  upper_len_var=metronome.stem_upper_var  upper_m=metronome.upper_mass  lower_m=metronome.lower_mass  b_pivot=metronome.b_pivot  esc_torque=metronome.esc_torque  t0_ang=-15 + (30)*rand(1,1)  t0_vel=metronome.initial_speed(3)
  M4 : sm_metronome_lib/M1  pivot_h=metronome.pivot_h  len=metronome.stem_length  upper_len=metronome.stem_upper  upper_len_var=metronome.stem_upper_var  upper_m=metronome.upper_mass  lower_m=metronome.lower_mass  b_pivot=metronome.b_pivot  esc_torque=metronome.esc_torque  t0_ang=-15 + (30)*rand(1,1)  t0_vel=metronome.initial_speed(4)
  Mux : Mux
  Simscape Bus1 : SimscapeBus  HierarchyStrings=M1;M2;M3;M4
  M : PMIOPort  Side=Left
  q : Outport
  wires:
  M3/1 -> Mux/3
  M1/1 -> Mux/1
  M2/1 -> Mux/2
  M4/1 -> Mux/4
  Mux/1 -> q/1
  connections:
  Simscape Bus1/RConn1 -- M/RConn1
  Simscape Bus1/LConn1 -- M1/LConn1
  Simscape Bus1/LConn2 -- M2/LConn1
  Simscape Bus1/LConn3 -- M3/LConn1
  Simscape Bus1/LConn4 -- M4/LConn1

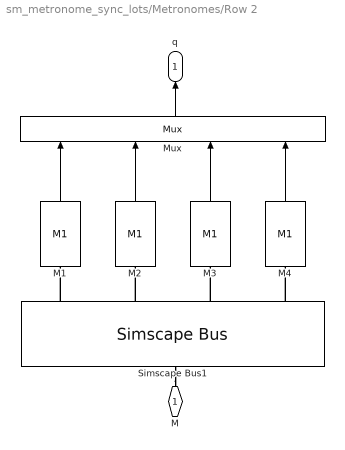
== system sm_metronome_sync_lots/Metronomes/Row 2 ==
  M1 : sm_metronome_lib/M1  pivot_h=metronome.pivot_h  len=metronome.stem_length  upper_len=metronome.stem_upper  upper_len_var=metronome.stem_upper_var  upper_m=metronome.upper_mass  lower_m=metronome.lower_mass  b_pivot=metronome.b_pivot  esc_torque=metronome.esc_torque  t0_ang=-15 + (30)*rand(1,1)  t0_vel=metronome.initial_speed(1)
  M2 : sm_metronome_lib/M1  pivot_h=metronome.pivot_h  len=metronome.stem_length  upper_len=metronome.stem_upper  upper_len_var=metronome.stem_upper_var  upper_m=metronome.upper_mass  lower_m=metronome.lower_mass  b_pivot=metronome.b_pivot  esc_torque=metronome.esc_torque  t0_ang=-15 + (30)*rand(1,1)  t0_vel=metronome.initial_speed(2)
  M3 : sm_metronome_lib/M1  pivot_h=metronome.pivot_h  len=metronome.stem_length  upper_len=metronome.stem_upper  upper_len_var=metronome.stem_upper_var  upper_m=metronome.upper_mass  lower_m=metronome.lower_mass  b_pivot=metronome.b_pivot  esc_torque=metronome.esc_torque  t0_ang=-15 + (30)*rand(1,1)  t0_vel=metronome.initial_speed(3)
  M4 : sm_metronome_lib/M1  pivot_h=metronome.pivot_h  len=metronome.stem_length  upper_len=metronome.stem_upper  upper_len_var=metronome.stem_upper_var  upper_m=metronome.upper_mass  lower_m=metronome.lower_mass  b_pivot=metronome.b_pivot  esc_torque=metronome.esc_torque  t0_ang=-15 + (30)*rand(1,1)  t0_vel=metronome.initial_speed(4)
  Mux : Mux
  Simscape Bus1 : SimscapeBus  HierarchyStrings=M1;M2;M3;M4
  M : PMIOPort  Side=Left
  q : Outport
  wires:
  Mux/1 -> q/1
  M4/1 -> Mux/4
  M2/1 -> Mux/2
  M1/1 -> Mux/1
  M3/1 -> Mux/3
  connections:
  Simscape Bus1/LConn4 -- M4/LConn1
  Simscape Bus1/LConn3 -- M3/LConn1
  Simscape Bus1/LConn2 -- M2/LConn1
  Simscape Bus1/LConn1 -- M1/LConn1
  Simscape Bus1/RConn1 -- M/RConn1

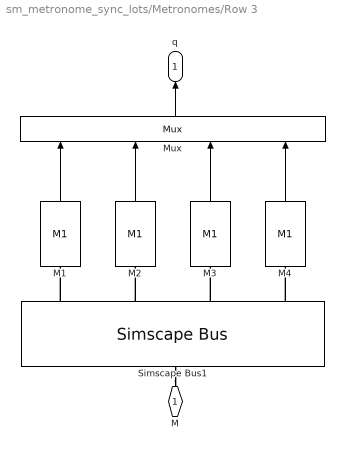
== system sm_metronome_sync_lots/Metronomes/Row 3 ==
  M1 : sm_metronome_lib/M1  pivot_h=metronome.pivot_h  len=metronome.stem_length  upper_len=metronome.stem_upper  upper_len_var=metronome.stem_upper_var  upper_m=metronome.upper_mass  lower_m=metronome.lower_mass  b_pivot=metronome.b_pivot  esc_torque=metronome.esc_torque  t0_ang=-15 + (30)*rand(1,1)  t0_vel=metronome.initial_speed(1)
  M2 : sm_metronome_lib/M1  pivot_h=metronome.pivot_h  len=metronome.stem_length  upper_len=metronome.stem_upper  upper_len_var=metronome.stem_upper_var  upper_m=metronome.upper_mass  lower_m=metronome.lower_mass  b_pivot=metronome.b_pivot  esc_torque=metronome.esc_torque  t0_ang=-15 + (30)*rand(1,1)  t0_vel=metronome.initial_speed(2)
  M3 : sm_metronome_lib/M1  pivot_h=metronome.pivot_h  len=metronome.stem_length  upper_len=metronome.stem_upper  upper_len_var=metronome.stem_upper_var  upper_m=metronome.upper_mass  lower_m=metronome.lower_mass  b_pivot=metronome.b_pivot  esc_torque=metronome.esc_torque  t0_ang=-15 + (30)*rand(1,1)  t0_vel=metronome.initial_speed(3)
  M4 : sm_metronome_lib/M1  pivot_h=metronome.pivot_h  len=metronome.stem_length  upper_len=metronome.stem_upper  upper_len_var=metronome.stem_upper_var  upper_m=metronome.upper_mass  lower_m=metronome.lower_mass  b_pivot=metronome.b_pivot  esc_torque=metronome.esc_torque  t0_ang=-15 + (30)*rand(1,1)  t0_vel=metronome.initial_speed(4)
  Mux : Mux
  Simscape Bus1 : SimscapeBus  HierarchyStrings=M1;M2;M3;M4
  M : PMIOPort  Side=Left
  q : Outport
  wires:
  Mux/1 -> q/1
  M4/1 -> Mux/4
  M2/1 -> Mux/2
  M1/1 -> Mux/1
  M3/1 -> Mux/3
  connections:
  Simscape Bus1/LConn4 -- M4/LConn1
  Simscape Bus1/LConn3 -- M3/LConn1
  Simscape Bus1/LConn2 -- M2/LConn1
  Simscape Bus1/LConn1 -- M1/LConn1
  Simscape Bus1/RConn1 -- M/RConn1

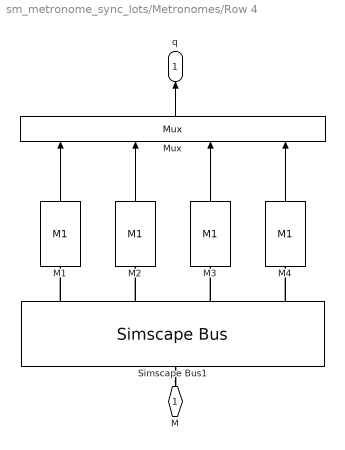
== system sm_metronome_sync_lots/Metronomes/Row 4 ==
  M1 : sm_metronome_lib/M1  pivot_h=metronome.pivot_h  len=metronome.stem_length  upper_len=metronome.stem_upper  upper_len_var=metronome.stem_upper_var  upper_m=metronome.upper_mass  lower_m=metronome.lower_mass  b_pivot=metronome.b_pivot  esc_torque=metronome.esc_torque  t0_ang=-15 + (30)*rand(1,1)  t0_vel=metronome.initial_speed(1)
  M2 : sm_metronome_lib/M1  pivot_h=metronome.pivot_h  len=metronome.stem_length  upper_len=metronome.stem_upper  upper_len_var=metronome.stem_upper_var  upper_m=metronome.upper_mass  lower_m=metronome.lower_mass  b_pivot=metronome.b_pivot  esc_torque=metronome.esc_torque  t0_ang=-15 + (30)*rand(1,1)  t0_vel=metronome.initial_speed(2)
  M3 : sm_metronome_lib/M1  pivot_h=metronome.pivot_h  len=metronome.stem_length  upper_len=metronome.stem_upper  upper_len_var=metronome.stem_upper_var  upper_m=metronome.upper_mass  lower_m=metronome.lower_mass  b_pivot=metronome.b_pivot  esc_torque=metronome.esc_torque  t0_ang=-15 + (30)*rand(1,1)  t0_vel=metronome.initial_speed(3)
  M4 : sm_metronome_lib/M1  pivot_h=metronome.pivot_h  len=metronome.stem_length  upper_len=metronome.stem_upper  upper_len_var=metronome.stem_upper_var  upper_m=metronome.upper_mass  lower_m=metronome.lower_mass  b_pivot=metronome.b_pivot  esc_torque=metronome.esc_torque  t0_ang=-15 + (30)*rand(1,1)  t0_vel=metronome.initial_speed(4)
  Mux : Mux
  Simscape Bus1 : SimscapeBus  HierarchyStrings=M1;M2;M3;M4
  M : PMIOPort  Side=Left
  q : Outport
  wires:
  M3/1 -> Mux/3
  M1/1 -> Mux/1
  M2/1 -> Mux/2
  M4/1 -> Mux/4
  Mux/1 -> q/1
  connections:
  Simscape Bus1/RConn1 -- M/RConn1
  Simscape Bus1/LConn1 -- M1/LConn1
  Simscape Bus1/LConn2 -- M2/LConn1
  Simscape Bus1/LConn3 -- M3/LConn1
  Simscape Bus1/LConn4 -- M4/LConn1
